simulink model "Observer_feedback"  (R2023a)
settings: Solver=VariableStepAuto  StartTime=0.0  StopTime=10.0  RelTol=1e-3
values from neighbouring files (symbols this model uses):
  A = [0 1 0 0 ; ((M+m)*g)/(M*L) 0 0 0; 0 0 0 1; (-m*g)/M 0 0 0]    [TP1.m]
  B = [0; -1/M*L;0;1/M]    [TP1.m]
  C = [1 0 0 0; 0 0 1 0]    [TP1.m]
  C_block = eye(4)    [TP1.m]
  D = [0;0;0;0]    [TP1.m]
  F = -place(A,B,p_desired)    [TP1.m]
  K_fast = place(A.',C.',p_fast).'    [TP1.m]
  x_0 = [0.1;0;0.1;0]    [TP1.m]
settings Model: Creator=jlancha2023  LastModifiedBy=jlancha2023
settings DataIOCC: Refine=4

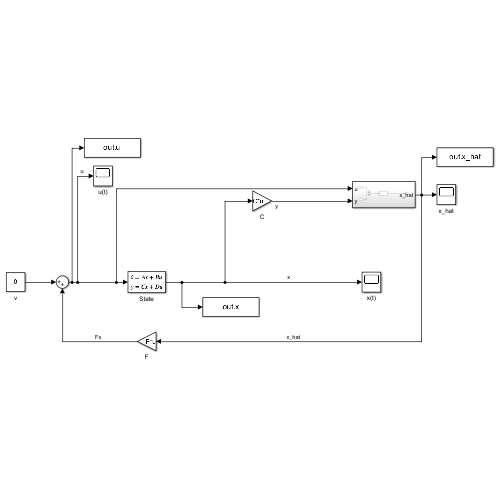
[thumbnail: Simulink's stored preview of the top-level diagram]
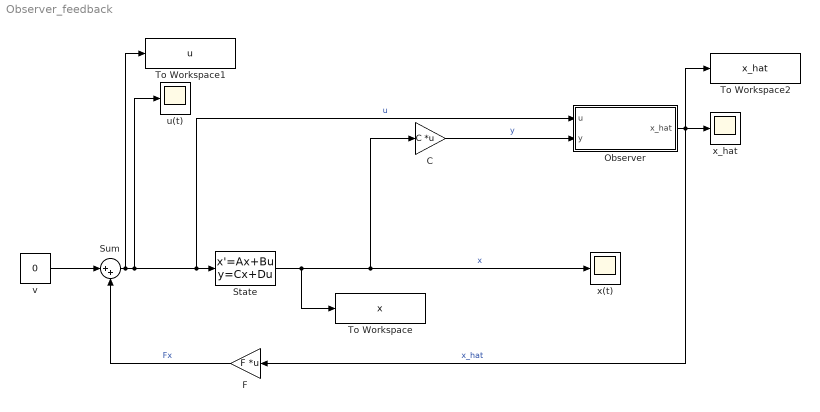
== system Observer_feedback ==
  C : Gain  Gain=C  Multiplication=Matrix(K*u)
  F : Gain  Gain=F  Multiplication=Matrix(K*u)
  Observer : Subsystem
  State : StateSpace  A=A  B=B  C=C_block  D=D  InitialCondition=x_0
  Sum : Sum  Inputs=|++
  To Workspace : ToWorkspace  VariableName=x  SampleTime=-1
  To Workspace1 : ToWorkspace  VariableName=u  SampleTime=-1
  To Workspace2 : ToWorkspace  VariableName=x_hat  SaveFormat=Timeseries  SampleTime=-1
  u(t) : Scope
  v : Constant  Value=0
  x(t) : Scope
  x_hat : Scope
  wires:
  Sum/1 -> Observer/1(u), State/1, u(t)/1, To Workspace1/1  "u"
  State/1 -> x(t)/1, C/1, To Workspace/1  "x"
  F/1 -> Sum/2  "Fx"
  v/1 -> Sum/1
  Observer/1(x_hat) -> To Workspace2/1, F/1, x_hat/1  "x_hat"
  C/1 -> Observer/2(y)  "y"

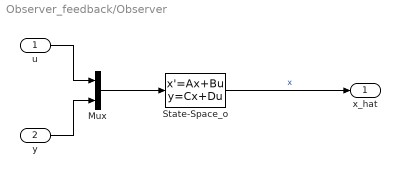
== system Observer_feedback/Observer ==
  u : Inport
  y : Inport  Port=2
  Mux : Mux  Inputs=2
  State-Space_o : StateSpace  A=A - K_fast*C  B=[B K_fast]  C=C_block  D=zeros(4,3)  InitialCondition=[0;0;0;0]
  x_hat : Outport
  wires:
  u/1 -> Mux/1
  y/1 -> Mux/2
  Mux/1 -> State-Space_o/1
  State-Space_o/1 -> x_hat/1  "x"
